simulink model "Integral_Action_Controller"  (R2020b)
settings: Solver=VariableStepAuto  StartTime=0.0  StopTime=5  RelTol=1e-3
model workspace (MAT data in the model file):
  A = [0  1  0  0; 0  -0.363636363636  2.67272727273  0; 0  0  0  1; 0  -0.909090909091  31.1818181818  0]
  B = [0; 1.81818181818; 0; 4.54545454545]
  C = Simulink.Parameter
  C.Value = [1  0  0  0; 0  1  0  0; 0  0  1  0; 0  0  0  1]
  C.DataType = 'auto'
  C.Dimensions = [4 4]
  D = [0; 0; 0; 0]
  Kc = Simulink.Parameter
  Kc.Value = [-150.1693 -65.2698 184.093 34.1629]
  Kc.DataType = 'auto'
  Kc.Dimensions = [1 4]
  Ki = Simulink.Parameter
  Ki.Value = 173.2051
  Ki.DataType = 'auto'
  Ki.Dimensions = [1 1]
settings Model: OrderedModelArguments=off  Creator=Alvaro  LastModifiedBy=Alvaro

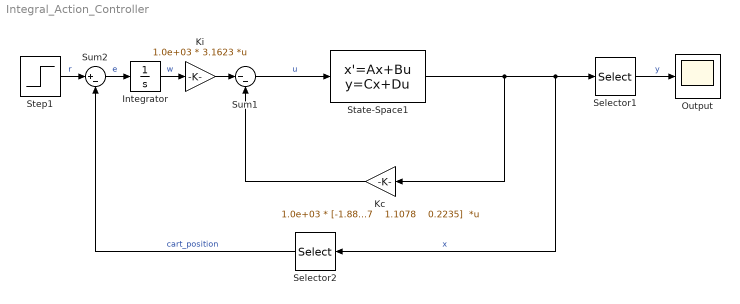
== system Integral_Action_Controller ==
  Integrator : Integrator
  Kc : Gain  Gain="1.0e+03 * [-1.8805   -0.5277    1.1078    0.2235]"  Multiplication=Matrix(K*u)
  Ki : Gain  Gain=1.0e+03 * 3.1623  Multiplication=Matrix(K*u)
  Output : Scope
  Selector1 : Selector  InputPortWidth=4  IndexOptions=Index vector (dialog)  Indices=[1 3]  OutputSizes=1
  Selector2 : Selector  InputPortWidth=4  IndexOptions=Index vector (dialog)  Indices=[1]  OutputSizes=1
  State-Space1 : StateSpace  A=A  B=B  C=C  D=D  InitialCondition=0
  Step1 : Step  Time=0.01  After=0.2  SampleTime=0.01
  Sum1 : Sum  Inputs=|--
  Sum2 : Sum  Inputs=|+-
  wires:
  Integrator/1 -> Ki/1  "w"
  Selector2/1 -> Sum2/2  "cart_position"
  Sum1/1 -> State-Space1/1  "u"
  Sum2/1 -> Integrator/1  "e"
  State-Space1/1 -> Selector1/1, Selector2/1, Kc/1  "x"
  Selector1/1 -> Output/1  "y"
  Step1/1 -> Sum2/1  "r"
  Kc/1 -> Sum1/2
  Ki/1 -> Sum1/1
